simulink model "SPWM"  (R2026a)
settings: Solver=VariableStepAuto  StopTime=2
undefined symbols (not defined in the file): Down, Up
libraries: eePwmGenerator x3, autolibpmsminterior x1
settings Model: Creator=mushen  LastModifiedBy=mushen

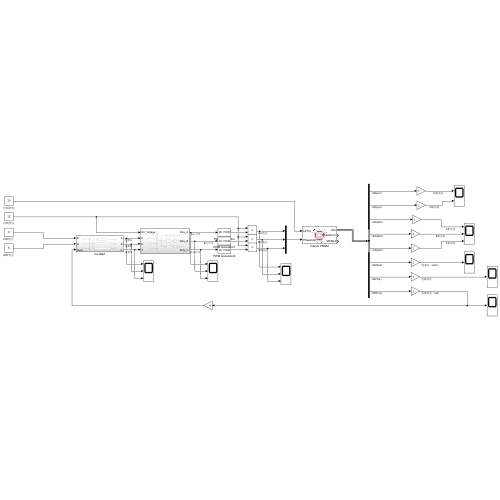
[thumbnail: Simulink's stored preview of the top-level diagram]
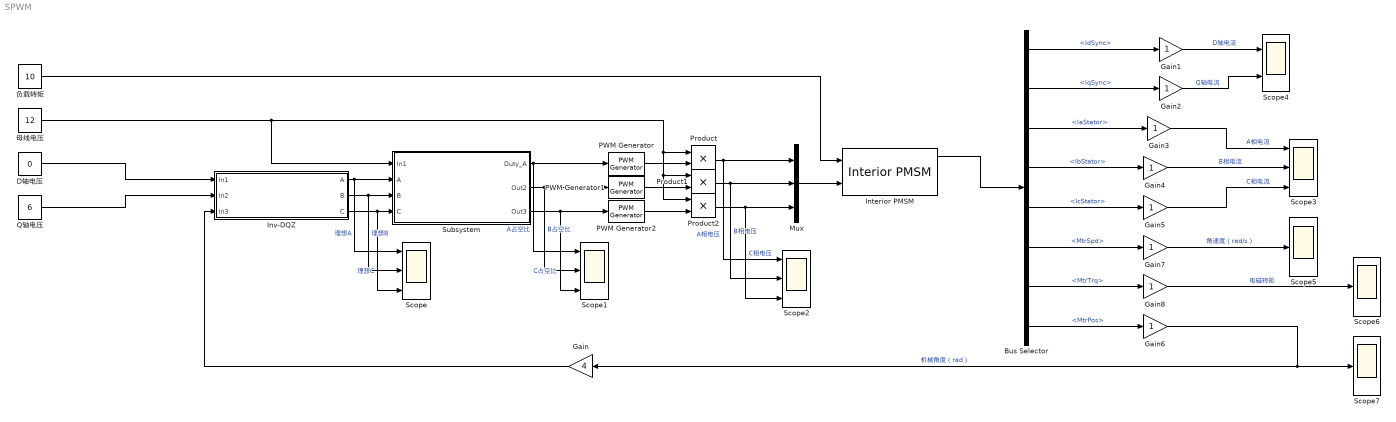
== system SPWM ==
  Bus Selector : BusSelector  OutputSignals=IdSync,IqSync,IaStator,IbStator,IcStator,MtrSpd,MtrTrq,MtrPos
  D轴电压 : Constant  Value=0
  Gain : Gain  Gain=4
  Gain{1..8} (8 alike) : Gain
  Interior PMSM : autolibpmsminterior/Interior PMSM  port_config=Torque  sim_type=Continuous  Ts=0.001  P=4  Rs=0.02  Ldq=[1.7e-3 3.2e-3]  KConstText=Permanent flux linkage constant (lambda_pm):  lambda_pm=0.2205  Ke=159.9771  mechanical=[0.002700,4.924e-4,0]  idq0=[0 0]  theta_init=0  omega_init=0  KConst=0.2205  lambda_pm_calc=0.2205  Kt=0.07  RefBlkName='autolibpmsminterior/Interior PMSM'  aMode=5
      settings: LibrarySourceBlock=mcblib/Electrical Systems/Motors/Interior PMSM
  Inv-DQZ : Subsystem
  Mux : Mux  Inputs=3
  PWM Generator : eePwmGenerator/PWM Generator  CarrCount=Up-Down  Tper=0.0001  Tdelay=0  Ts=5e-6
  PWM Generator1 : eePwmGenerator/PWM Generator  CarrCount=Up-Down  Tper=0.0001  Tdelay=0  Ts=5e-6
  PWM Generator2 : eePwmGenerator/PWM Generator  CarrCount=Up-Down  Tper=0.0001  Tdelay=0  Ts=5e-6
  Product : Product
  Product1 : Product
  Product2 : Product
  Q轴电压 : Constant  Value=6
  Scope{,1..3} (4 alike) : Scope  NumInputPorts=3
      Scope settings: ActiveDisplayYMinimum=-7.4999999999542695  ActiveDisplayYMaximum=7.49999999991693
      Scope1 settings: ActiveDisplayYMinimum=-0.12499999999618908  ActiveDisplayYMaximum=1.1249999999930773
      Scope2 settings: ActiveDisplayYMinimum=-1.4999999999999996  ActiveDisplayYMaximum=13.5  DataLoggingVariableName=ScopeData2
      Scope3 settings: ActiveDisplayYMinimum=-42.298704643275528  ActiveDisplayYMaximum=42.305828836843332  DataLoggingVariableName=ScopeData3
  Scope4 : Scope  NumInputPorts=2
      settings: ActiveDisplayYMinimum=-7.4999999999542695  ActiveDisplayYMaximum=7.49999999991693  DataLoggingVariableName=ScopeData4
  Scope5 : Scope
      settings: ActiveDisplayYMinimum=-8.3500269440904287  ActiveDisplayYMaximum=20.77178175547505  DataLoggingVariableName=ScopeData5
  Scope6 : Scope
      settings: ActiveDisplayYMinimum=-7.4999999999542695  ActiveDisplayYMaximum=7.49999999991693  DataLoggingVariableName=ScopeData6
  Scope7 : Scope
      settings: ActiveDisplayYMinimum=-7.4999999999542695  ActiveDisplayYMaximum=7.49999999991693  DataLoggingVariableName=ScopeData7
  Subsystem : Subsystem
  母线电压 : Constant  Value=12
  负载转矩 : Constant  Value=10
  wires:
  Subsystem/2(Out2) -> Scope1/2, PWM Generator1/1  "B占空比"
  Inv-DQZ/2(B) -> Scope/2, Subsystem/3(B)  "理想B"
  PWM Generator1/1 -> Product1/2
  Product1/1 -> Scope2/2, Mux/2  "B相电压"
  Product/1 -> Scope2/1, Mux/1  "A相电压"
  PWM Generator2/1 -> Product2/2
  D轴电压/1 -> Inv-DQZ/1(In1)
  母线电压/1 -> Product2/1, Product1/1, Product/1, Subsystem/1(In1)
  Subsystem/3(Out3) -> Scope1/3, PWM Generator2/1  "C占空比"
  Subsystem/1(Duty_A) -> Scope1/1, PWM Generator/1  "A占空比"
  Inv-DQZ/3(C) -> Scope/3, Subsystem/4(C)  "理想C"
  Product2/1 -> Mux/3, Scope2/3  "C相电压"
  Q轴电压/1 -> Inv-DQZ/2(In2)
  PWM Generator/1 -> Product/2
  Inv-DQZ/1(A) -> Scope/1, Subsystem/2(A)  "理想A"
  Gain/1 -> Inv-DQZ/3(In3)
  Mux/1 -> Interior PMSM/2
  Bus Selector/8 -> Gain6/1  "<MtrPos>"
  Bus Selector/1 -> Gain1/1  "<IdSync>"
  Bus Selector/2 -> Gain2/1  "<IqSync>"
  Gain1/1 -> Scope4/1  "D轴电流"
  Gain2/1 -> Scope4/2  "Q轴电流"
  Gain5/1 -> Scope3/3  "C相电流"
  Gain4/1 -> Scope3/2  "B相电流"
  Gain3/1 -> Scope3/1  "A相电流"
  Bus Selector/3 -> Gain3/1  "<IaStator>"
  Bus Selector/4 -> Gain4/1  "<IbStator>"
  Bus Selector/5 -> Gain5/1  "<IcStator>"
  Bus Selector/6 -> Gain7/1  "<MtrSpd>"
  负载转矩/1 -> Interior PMSM/1
  Gain6/1 -> Gain/1, Scope7/1  "机械角度（rad）"
  Gain7/1 -> Scope5/1  "角速度（rad/s）"
  Bus Selector/7 -> Gain8/1  "<MtrTrq>"
  Gain8/1 -> Scope6/1  "电磁转矩"
  Interior PMSM/1 -> Bus Selector/1

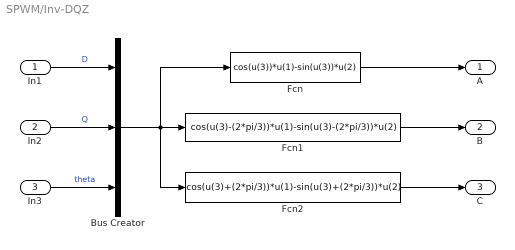
== system SPWM/Inv-DQZ ==
  In1 : Inport
  In2 : Inport  Port=2
  In3 : Inport  Port=3
  Bus Creator : BusCreator  Inputs=3
  Fcn : Fcn  Expr=cos(u(3))*u(1)-sin(u(3))*u(2)
  Fcn1 : Fcn  Expr=cos(u(3)-(2*pi/3))*u(1)-sin(u(3)-(2*pi/3))*u(2)
  Fcn2 : Fcn  Expr=cos(u(3)+(2*pi/3))*u(1)-sin(u(3)+(2*pi/3))*u(2)
  A : Outport
  B : Outport  Port=2
  C : Outport  Port=3
  wires:
  In3/1 -> Bus Creator/3  "theta"
  In2/1 -> Bus Creator/2  "Q"
  In1/1 -> Bus Creator/1  "D"
  Bus Creator/1 -> Fcn/1, Fcn1/1, Fcn2/1
  Fcn/1 -> A/1
  Fcn1/1 -> B/1
  Fcn2/1 -> C/1

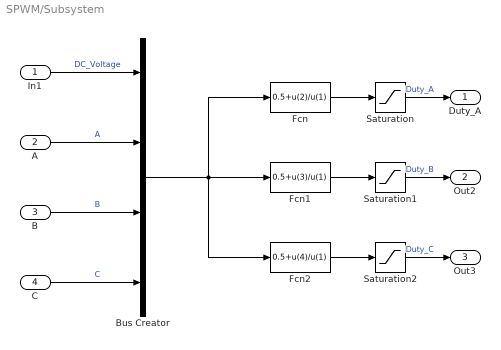
== system SPWM/Subsystem ==
  In1 : Inport
  A : Inport  Port=2
  B : Inport  Port=3
  C : Inport  Port=4
  Bus Creator : BusCreator  Inputs=4
  Fcn : Fcn  Expr=0.5+u(2)/u(1)
  Fcn1 : Fcn  Expr=0.5+u(3)/u(1)
  Fcn2 : Fcn  Expr=0.5+u(4)/u(1)
  Saturation : Saturate  UpperLimit=1  LowerLimit=0
  Saturation1 : Saturate  UpperLimit=1  LowerLimit=0
  Saturation2 : Saturate  UpperLimit=1  LowerLimit=0
  Duty_A : Outport
  Out2 : Outport  Port=2
  Out3 : Outport  Port=3
  wires:
  In1/1 -> Bus Creator/1  "DC_Voltage"
  A/1 -> Bus Creator/2  "A"
  B/1 -> Bus Creator/3  "B"
  C/1 -> Bus Creator/4  "C"
  Fcn/1 -> Saturation/1
  Bus Creator/1 -> Fcn/1, Fcn2/1, Fcn1/1
  Saturation/1 -> Duty_A/1  "Duty_A"
  Saturation1/1 -> Out2/1  "Duty_B"
  Fcn1/1 -> Saturation1/1
  Saturation2/1 -> Out3/1  "Duty_C"
  Fcn2/1 -> Saturation2/1
